simulink model "e_bike"  (R2019b)
settings: Solver=VariableStepAuto  StartTime=0.0  StopTime=1000  RelTol=1e-3
InitFcn:
  | Rho_air= 1.225;
  | C_d=0.9;
  | A_d= 0.4;
  | Static_Friction_Coefficient =0.0015;
  | Dynamic_Friction_Coefficient= 0.0015;
  | Cyclist_weight=85;
  | Vehicle_mass = 25;
  | g = 9.81;
  | Wheel_mass = 0.25;
  | Tire_mass = 0.25;
  | Abs = 1;
  | Bb=0.2;
  | Wheel_Radius = 0.3;
  | F_Rider = 100;
  | Wheel_Inertia=0.0225;
  | Braking_Pressure=100;
  | Crank_Length = 0.150;
  | Angle_of_crank = [0:1:360;0:1:360;]';
  | Number_of_brake_pad = 2;
  | Coefficient_of_Brake_friction = 0.9;
  | Effective_Radius_of_Disc = 0.16;
  | Outer_Radius_of_Brake = 0.18;
  | Inner_Radius_of_Brake = 0.14;
  | Disc_Mass=0;
  | Heat_capacity=0;
  | Surface_Temp=0;
  | Ambient_Temp=0;
  | Thermal_Conductivity=1;
  | 
  | Motor_torque_constant = 0.75; % NM/A
  | Kb = (51.7/(1000*2*pi/60)); %or  V/Wm (wm in rps) volt/rps
  | Jm =10.2 *10^-3; %kgm^2
  | Bm = ((Motor_torque_constant)*(17)/(1000*2*pi/60));
  | Motor_resistance =88*10^-2; %ohm
  | L = 0.36*10^-3;% H(henry)
  | alpha_Conductor =0.0040;
  | Ref_Temp = 25;
  | Alpha_Magnet = -0.0020;
  | 
  | Internal_Resistance =95*10^-3; %ohm
  | capacity =19.5 ; %Ah
  | SOC_initial = 100;
  | Polarization_Resistance = 95*10^-3;
  | Polarization_Capacitance = 1*10^-7;
undefined symbols (not defined in the file or in its folder): V
libraries: simulink x2
(part 3 of 3)

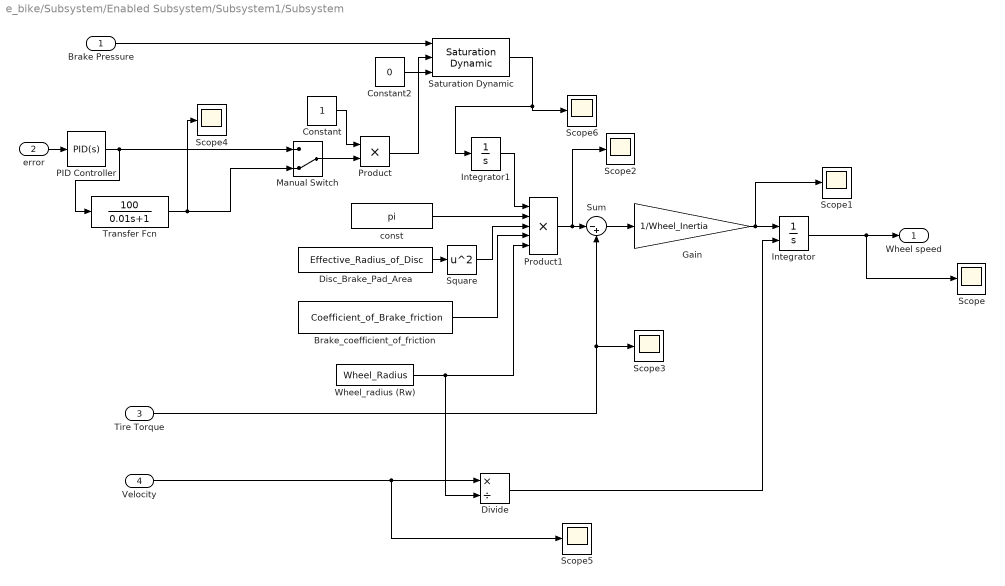
== system e_bike/Subsystem/Enabled Subsystem/Subsystem1/Subsystem ==
  Brake Pressure : Inport
  "error " : Inport  Port=2
  Tire Torque : Inport  Port=3
  Velocity : Inport  Port=4
  Brake_coefficient_of_friction : Constant  Value=Coefficient_of_Brake_friction
  Constant : Constant
  Constant2 : Constant  Value=0
  Disc_Brake_Pad_Area : Constant  Value=Effective_Radius_of_Disc
  Divide : Product  Inputs=*/
  Gain : Gain  Gain=1/Wheel_Inertia
  Integrator : Integrator  InitialConditionSource=external  InitialCondition=V/Wheel_Radius  LimitOutput=on  UpperSaturationLimit=1000  LowerSaturationLimit=0
  Integrator1 : Integrator  UpperSaturationLimit=Braking_Pressure
  Manual Switch : ManualSwitch  CurrentSetting=0
  PID Controller : simulink/Continuous/PID Controller  Controller=PID  Form=Parallel  TimeDomain=Continuous-time  SampleTime=-1  IntegratorMethod=Forward Euler  FilterMethod=Forward Euler  ControllerParametersSource=internal  P=22  I=4  D=0.4  UseFilter=on  N=100  TunerSelectOption=Transfer Function Based (PID Tuner App)  InitialConditionSource=internal  InitialConditionForIntegrator=0  InitialConditionForFilter=0  DifferentiatorICPrevScaledInput=0  ExternalReset=none  TrackingMode=off  Kt=1  LimitOutput=off  UpperSaturationLimit=inf  LowerSaturationLimit=-inf  LinearizeAsGain=on  AntiWindupMode=none  Kb=1  POutMin=[]  POutMax=[]  IOutMin=[]  IOutMax=[]  DOutMin=[]  DOutMax=[]  NOutMin=[]  NOutMax=[]  SumOutMin=[]  SumOutMax=[]  SaturationOutMin=[]  SaturationOutMax=[]  PParamMin=[]  PParamMax=[]  IParamMin=[]  IParamMax=[]  DParamMin=[]  DParamMax=[]  NParamMin=[]  NParamMax=[]  KbParamMin=[]  KbParamMax=[]  KtParamMin=[]  KtParamMax=[]  KbOutMin=[]  KbOutMax=[]  KtOutMin=[]  KtOutMax=[]  IntegratorOutMin=[]  IntegratorOutMax=[]  FilterOutMin=[]  FilterOutMax=[]  SumI1OutMin=[]  SumI1OutMax=[]  SumI2OutMin=[]  SumI2OutMax=[]  SumI3OutMin=[]  SumI3OutMax=[]  SumI4OutMin=[]  SumI4OutMax=[]  SumDOutMin=[]  SumDOutMax=[]  DifferentiatorOutMin=[]  DifferentiatorOutMax=[]  FilterDiffOutCoefMin=[]  FilterDiffOutCoefMax=[]  ReciprocalOutMin=[]  ReciprocalOutMax=[]  SumDenOutMin=[]  SumDenOutMax=[]  SumNumOutMin=[]  SumNumOutMax=[]  DivideOutMin=[]  DivideOutMax=[]  IntegratorContinuousStateAttributes=''  IntegratorStateMustResolveToSignalObject=off  IntegratorRTWStateStorageClass=Auto  FilterContinuousStateAttributes=''  FilterStateMustResolveToSignalObject=off  FilterRTWStateStorageClass=Auto  ParallelPVariant=InternalParameters  IdealPVariant=Disabled  IVariant=InternalParameters  DVariant=InternalParameters  IntegratorVariant=Continuous  SatVariant=Disabled  AWVariant=Passthrough  PCopyVariant=Disabled  TRVariant=Disabled  FdbkBlocksVariant=Forward  IdealPFdbkVariant=Disabled  SatFdbkVariant=Disabled  DerivativeFilterVariant=ContFilter  NVariant=InternalParameters  NCopyVariant=Disabled  FilterICVariant=InternalICsFilter  IntegratorICVariant=InternalICs  ExternalResetVariant=Disabled  TRSumVariant=Passthrough  SumFdbkVariant=Disabled  SumVariant=Sum_PID
  Product : Product
  Product1 : Product  Inputs=5
  Saturation Dynamic : simulink/Discontinuities/Saturation Dynamic  OutMin=[]  OutMax=[]  OutDataTypeStr=Inherit: Same as second input  OutDataType=fixdt(1, 16)  OutScaling=2^-10  DoSatur=off
  Scope{,1..6} (7 alike) : Scope
  Square : Math  Operator=square  SaturateOnIntegerOverflow=on
  Sum : Sum  Inputs=|-+
  Transfer Fcn : TransferFcn  Numerator=[100]  Denominator=[0.01 1]
  "Wheel_radius (Rw) " : Constant  Value=Wheel_Radius
  "const " : Constant  Value=pi
  "Wheel speed " : Outport
  wires:
  "error "/1 -> PID Controller/1
  Constant/1 -> Product/1
  "const "/1 -> Product1/2
  Disc_Brake_Pad_Area/1 -> Square/1
  Square/1 -> Product1/3
  Brake_coefficient_of_friction/1 -> Product1/4
  Product1/1 -> Scope2/1, Sum/1
  Tire Torque/1 -> Scope3/1, Sum/2
  Sum/1 -> Gain/1
  Gain/1 -> Scope1/1, Integrator/1
  Manual Switch/1 -> Product/2
  PID Controller/1 -> Transfer Fcn/1, Manual Switch/1
  Integrator1/1 -> Product1/1
  Velocity/1 -> Scope5/1, Divide/1
  Divide/1 -> Integrator/2
  "Wheel_radius (Rw) "/1 -> Divide/2, Product1/5
  Integrator/1 -> "Wheel speed "/1, Scope/1
  Transfer Fcn/1 -> Scope4/1, Manual Switch/2
  Constant2/1 -> Saturation Dynamic/3
  Product/1 -> Saturation Dynamic/2
  Saturation Dynamic/1 -> Scope6/1, Integrator1/1
  Brake Pressure/1 -> Saturation Dynamic/1

== stateflow chart e_bike/Subsystem/Chart ==
  (junction 5) -> (junction 9) : {signal=1}
  (junction 2) -> (junction 5) [order 1] : [u>725]
  (junction 9) -> (junction 15)
  (default) -> (junction 2)
  (junction 15) -> (junction 18)
  (junction 2) -> (junction 7) [order 2] : [u<725]
  (junction 13) -> (junction 15)
  (junction 7) -> (junction 13) : {signal=0}
  data: u input; signal output

== stateflow chart e_bike/Environmental_Subsystem/Chart ==
  (junction 5) -> (junction 9) : {signal=1}
  (junction 2) -> (junction 5) [order 1] : [u>0]
  (junction 9) -> (junction 15)
  (default) -> (junction 2)
  (junction 15) -> (junction 18)
  (junction 2) -> (junction 7) [order 2] : [u==0]
  (junction 13) -> (junction 15)
  (junction 7) -> (junction 13) : {signal=0}
  data: u input; signal output
